simulink model "Problem_1"  (R2020a)
settings: Solver=VariableStepAuto  StartTime=0.0  StopTime=10.0  RelTol=1e-3
PreLoadFcn:
  | m1=100;
  | k1=50;
  | b=50;
  | k2=25;
  | m2=4;
settings Model: Creator=Ganesh  LastModifiedBy=Avengers

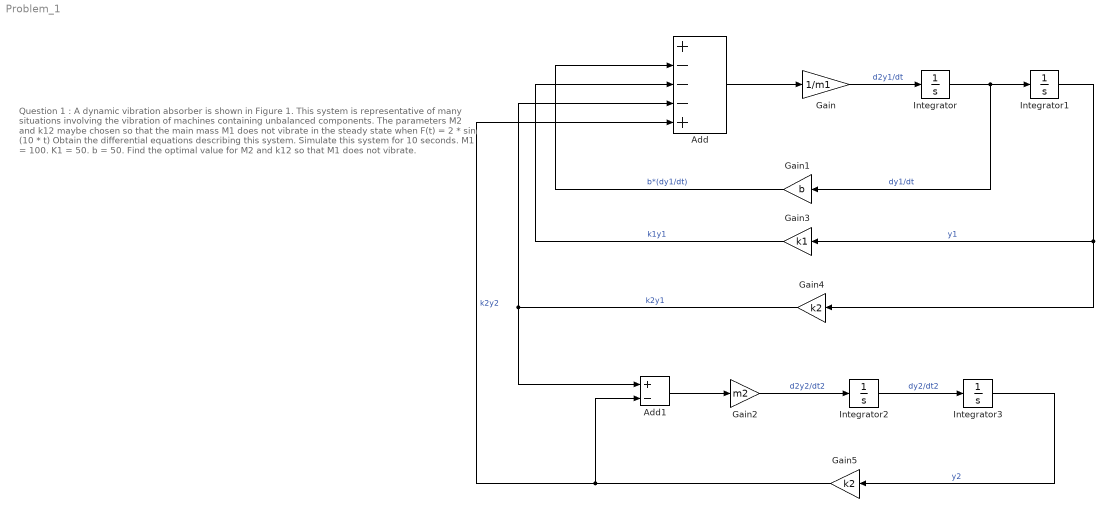
== system Problem_1 ==
  note: Question 1 :
      | A dynamic vibration absorber is shown in Figure 1. This system is representative of many situations involving the vibration of machines containing unbalanced components. The parameters M2 and k12 maybe chosen so that the main mass M1 does not vibrate in the steady state when F(t) = 2 * sin (10 * t)
      | Obtain the differential equations describing this system.
      | Simulate this system for 10 seconds. M1 = 100. K1 = 50. b = 50.
      | Find the optimal value for M2 and k12 so that M1 does not vibrate.
  Add : Sum  Inputs=+---+
  Add1 : Sum  Inputs=+-
  Gain : Gain  Gain=1/m1
  Gain1 : Gain  Gain=b
  Gain2 : Gain  Gain=m2
  Gain3 : Gain  Gain=k1
  Gain4 : Gain  Gain=k2
  Gain5 : Gain  Gain=k2
  Integrator{,1..3} (4 alike) : Integrator
  wires:
  Gain/1 -> Integrator/1  "d2y1/dt"
  Gain1/1 -> Add/2  "b*(dy1/dt)"
  Add/1 -> Gain/1
  Integrator/1 -> Gain1/1, Integrator1/1  "dy1/dt"
  Integrator1/1 -> Gain4/1, Gain3/1  "y1"
  Gain3/1 -> Add/3  "k1y1"
  Gain4/1 -> Add1/1, Add/4  "k2y1"
  Add1/1 -> Gain2/1
  Gain2/1 -> Integrator2/1  "d2y2/dt2"
  Integrator2/1 -> Integrator3/1  "dy2/dt2"
  Integrator3/1 -> Gain5/1  "y2"
  Gain5/1 -> Add1/2, Add/5  "k2y2"
